simulink model "sltestThrottlePositionSensorMdlRef"  (R2023a)
settings: Solver=FixedStepDiscrete  StartTime=0.0  StopTime=10.0  FixedStep=0.005  RelTol=1e-3
PreLoadFcn:
  | TPSPercent_LkupTbl = Simulink.LookupTable;
  | TPSPercent_LkupTbl.Table.DataType = 'single';
  | TPSPercent_LkupTbl.Table.Min = [];
  | TPSPercent_LkupTbl.Table.Max = [];
  | TPSPercent_LkupTbl.Table.Unit = '';
  | TPSPercent_LkupTbl.Table.FieldName = 'Table';
  | TPSPercent_LkupTbl.Table.Description = '';
  | TPSPercent_LkupTbl.Table.Value = ...
  |   [0 10 20 30 40 50 60 70 80 90 100];
  | TPSPercent_LkupTbl.BreakpointsSpecification = 'Explicit values';
  | TPSPercent_LkupTbl.SupportTunableSize = false;
  | TPSPercent_LkupTbl.Breakpoints.DataType = 'single';
  | TPSPercent_LkupTbl.Breakpoints.Min = [];
  | TPSPercent_LkupTbl.Breakpoints.Max = [];
  | TPSPercent_LkupTbl.Breakpoints.Unit = '';
  | TPSPercent_LkupTbl.Breakpoints.FieldName = 'BP1';
  | TPSPercent_LkupTbl.Breakpoints.Description = '';
  | TPSPercent_LkupTbl.Breakpoints.Value = ...
  |   [0 100 200 300 400 500 600 700 800 900 1000];
  | TPSPercent_LkupTbl.Breakpoints.TunableSizeName = 'N1';
  | TPSPercent_LkupTbl.CoderInfo.StorageClass = 'Auto';
  | TPSPercent_LkupTbl.StructTypeInfo.Name = 'MyStruct';
  | TPSPercent_LkupTbl.StructTypeInfo.DataScope = 'Auto';
  | TPSPercent_LkupTbl.StructTypeInfo.HeaderFileName = '';
undefined symbols (not defined in the file): TPSPercentBkpt, TPSPercentTbl
settings Model: Creator=The MathWorks, Inc.  LastModifiedBy=The MathWorks, Inc.
settings SolverCC: AlgebraicLoopSolver=TrustRegion  MaxZcPerStep=1
settings DataIOCC: SaveFormat=StructureWithTime  ReturnWorkspaceOutputs=off
settings OptimizationCC: DefaultParameterBehavior=Inlined  PassReuseOutputArgsAs=Individual arguments  ZeroExternalMemoryAtStartup=off  ZeroInternalMemoryAtStartup=off  EfficientTunableParamExpr=on
settings DebuggingCC: ParameterTunabilityLossMsg=error  UnconnectedInputMsg=warning  UnconnectedOutputMsg=warning  UnconnectedLineMsg=warning  ArithmeticOperatorsInVariantConditions=warning
settings ModelReferenceCC: EnableRefExpFcnMdlSchedulingChecks=on
settings SFSimCC: SimUseLocalCustomCode=off  MATLABDynamicMemAlloc=off  CustomCodeUndefinedFunction=UseInterfaceOnly
settings RTWCC: Description=AUTOSAR  SystemTargetFile=autosar.tlc  GenCodeOnly=on  TemplateMakefile=ert_default_tmf  GenerateReport=on  RTWUseLocalCustomCode=off  IncludeHyperlinkInReport=on  LaunchReport=on  PortableWordSizes=on  GenerateTraceInfo=on  GenerateTraceReport=on  GenerateTraceReportSl=on  GenerateTraceReportSf=on  GenerateTraceReportEml=on  DLArmComputeVersion=19.05
settings CodeAppCC: ForceParamTrailComments=on  IgnoreCustomStorageClasses=off  OperatorAnnotations=on  SimulinkDataObjDesc=on  SFDataObjDesc=on  InsertBlockDesc=on
settings STFCustomTargetCC: MultiwordLength=256  ParMdlRefBuildCompliant=on  CompOptLevelCompliant=on  ConcurrentExecutionCompliant=off  IncludeMdlTerminateFcn=off  CombineOutputUpdateFcns=on  SuppressErrorStatus=on  ERTCustomFileBanners=on  CodeInterfacePackaging=Reusable function  SupportNonFinite=off  SupportComplex=off  SupportContinuousTime=off  SupportNonInlinedSFcns=off  RemoveResetFunc=on  MATLABClassNameForMDSCustomization=Simulink.SoftwareTarget.ERTCustomization  AutosarCompliant=on  GRTInterface=off  LookupTableObjectStructAxisOrder=2,1,3,4,...  LUTObjectStructOrderEvenSpacing=Size,Table,Breakpoints  SystemTargetFile=autosar.tlc
settings ERTTargetCC: TargetLangStandard=C99 (ISO)  ConcurrentExecutionCompliant=off  IncludeMdlTerminateFcn=off  SuppressErrorStatus=on  CodeInterfacePackaging=Reusable function  SupportNonFinite=off  SupportComplex=off  ModelStepFunctionPrototypeControlCompliant=off  CPPClassGenCompliant=off  AutosarCompliant=on  LookupTableObjectStructAxisOrder=2,1,3,4,...  LUTObjectStructOrderEvenSpacing=Size,Table,Breakpoints  InlinedParameterPlacement=NonHierarchical  ERTCustomFileTemplate=example_file_process.tlc

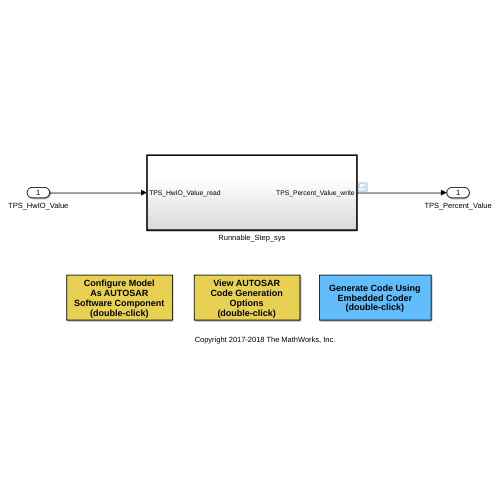
[thumbnail: Simulink's stored preview of the top-level diagram]
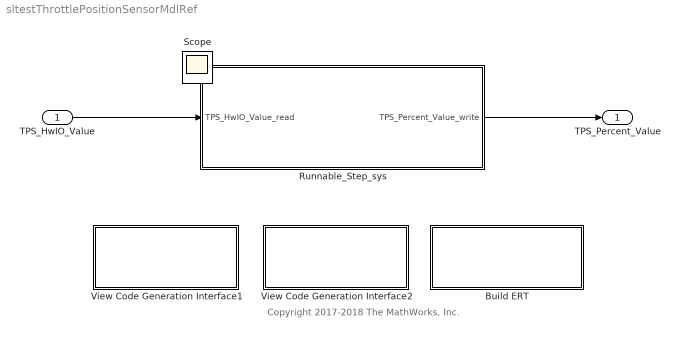
== system sltestThrottlePositionSensorMdlRef ==
  note: Copyright 2017-2018 The MathWorks, Inc.
  TPS_HwIO_Value : Inport  OutDataTypeStr=uint16  PortDimensions=1
  Build ERT : Subsystem  mask{attrib_overrides={'RTWCAPIParams','RTWCAPISignals','RTWCAPIStates'}}
      mask prompts: attrib_overrides "List of attributes to preserve (cell of strings):"
      mask help: Enter the attributes of the configuration set that you want preserved. Otherwise, the default configuration script will override your current settings.
      settings: OpenFcn=|
      | try
      |     if ~exist('rtwdemo_ert', 'dir')
      |         disp('Creating working directory rtwdemo_ert')
      |         mkdir('rtwdemo_ert')
      |     end
      |     cd('rtwdemo_ert');
      |     rtwbuilddemomodel(bdroot);
      |     cd('..');
      | catch myException
      |     rethrow(myException);
      | end
      mask Display:
      | disp(['Generate Code Using\n',...
      | 	 'Embedded Coder\n'...
      | 	  '(double-click)'])
  Runnable_Step_sys : Subsystem  TreatAsAtomicUnit=on  SystemSampleTime=0.005
  View Code Generation Interface1 : Subsystem
      settings: OpenFcn=autosar_ui_launch(bdroot)
      mask Display: disp('Configure Model\nAs AUTOSAR\nSoftware Component\n(double-click)')
  View Code Generation Interface2 : Subsystem
      settings: OpenFcn=|
      | dlg = slCfgPrmDlg(bdroot,'Open');
      | dlg = slCfgPrmDlg(bdroot,'TurnToPage',[message('RTW:configSet:configSetCodeGen').getString,'/',message('RTW:autosar:autosarCodeGenOptions').getString]);
      | clear dlg;
      mask Display: disp('View AUTOSAR\nCode Generation\nOptions\n(double-click)')
  TPS_Percent_Value : Outport  OutDataTypeStr=single  PortDimensions=1  VectorParamsAs1DForOutWhenUnconnected=off
  Scope : Scope
  wires:
  TPS_HwIO_Value/1 -> Runnable_Step_sys/1(TPS_HwIO_Value_read)
  Runnable_Step_sys/1(TPS_Percent_Value_write) -> TPS_Percent_Value/1

== system sltestThrottlePositionSensorMdlRef/Build ERT ==

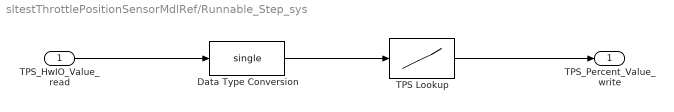
== system sltestThrottlePositionSensorMdlRef/Runnable_Step_sys ==
  TPS_HwIO_Value_read : Inport
  Data Type Conversion : DataTypeConversion  OutDataTypeStr=single  SaturateOnIntegerOverflow=off  RndMeth=Floor
  TPS Lookup : Lookup_n-D  NumberOfTableDimensions=1  DataSpecification=Lookup table object  LookupTableObject=TPSPercent_LkupTbl  BreakpointsForDimension1=TPSPercentBkpt  BreakpointsForDimension1DataTypeStr=single  IndexSearchMethod=Linear search  Table=TPSPercentTbl  TableDataTypeStr=single  ExtrapMethod=Clip  InternalRulePriority=Speed  OutDataTypeStr=single  RndMeth=Simplest
  TPS_Percent_Value_write : Outport  VectorParamsAs1DForOutWhenUnconnected=off
  wires:
  TPS_HwIO_Value_read/1 -> Data Type Conversion/1
  TPS Lookup/1 -> TPS_Percent_Value_write/1
  Data Type Conversion/1 -> TPS Lookup/1

== system sltestThrottlePositionSensorMdlRef/View Code Generation Interface1 ==

== system sltestThrottlePositionSensorMdlRef/View Code Generation Interface2 ==
